simulink model "Template_v3_08_2022a_Jetson"  (R2022a)
settings: Solver=FixedStepAuto  StartTime=0.0  StopTime=tsim  FixedStep=baseRate  RelTol=1e-3  EnableMultiTasking=on
values from neighbouring files (symbols this model uses):
  baseRate = 0.05    [Run_Initializer.m]
  drop_states_ARM = [ pi/2, pi/2, 0]    [Run_Initializer.m]
  drop_states_BLACK = [ xLength/2, yLength/2, 0]    [Run_Initializer.m]
  drop_states_BLUE = [ xLength/2-0.5; yLength/2; 0]    [Run_Initializer.m]
  drop_states_RED = [ xLength/2+0.5, yLength/2, pi]    [Run_Initializer.m]
  F_Black_X_nominal = 0.2196    [Run_Initializer.m]
  F_Black_Y_nominal = 0.2825    [Run_Initializer.m]
  F_Blue_X_nominal = 0.2196    [Run_Initializer.m]
  F_Blue_Y_nominal = 0.2825    [Run_Initializer.m]
  F_red_X_nominal = 0.2196    [Run_Initializer.m]
  F_red_Y_nominal = 0.2825    [Run_Initializer.m]
  F_thrusters_BLACK = [F_Black_X_nominal; F_Black_X_nominal;                             F_Black_Y_nominal; F_Black_Y_nominal; F_Black_X_nominal;                              F_Black_X_nominal; F_Black_Y_nominal; F_Black_Y_nominal]    [Run_Initializer.m]
  F_thrusters_BLUE = [F_Blue_X_nominal; F_Blue_X_nominal;                             F_Blue_Y_nominal; F_Blue_Y_nominal; F_Blue_X_nominal;                              F_Blue_X_nominal; F_Blue_Y_nominal; F_Blue_Y_nominal]    [Run_Initializer.m]
  F_thrusters_RED = [F_red_X_nominal; F_red_X_nominal;                             F_red_Y_nominal; F_red_Y_nominal; F_red_X_nominal;                              F_red_X_nominal; F_red_Y_nominal; F_red_Y_nominal]    [Run_Initializer.m]
  Gamma1 = 0.0025    [Run_Initializer.m]
  Gamma2 = 100    [Run_Initializer.m]
  Gamma3 = 10    [Run_Initializer.m]
  Gamma4 = 0.001    [Run_Initializer.m]
  Gamma5 = 100    [Run_Initializer.m]
  Gamma6 = 0.001    [Run_Initializer.m]
  home_states_BLACK = [ xLength/2; yLength/2; 0]    [Run_Initializer.m]
  home_states_BLUE = [ xLength/2-0.9; yLength/2; 0]    [Run_Initializer.m]
  home_states_RED = [ xLength/2+0.9; yLength/2; pi]    [Run_Initializer.m]
  init_states_BLACK = [ xLength/2; yLength/2; 0]    [Run_Initializer.m]
  init_states_BLUE = [ xLength/2-0.9; yLength/2; 0]    [Run_Initializer.m]
  init_states_RED = [ xLength/2+0.9; yLength/2; pi]    [Run_Initializer.m]
  Kd_elarm = 0.05    [Run_Initializer.m]
  Kd_sharm = 0.05    [Run_Initializer.m]
  Kd_tb = 0.4    [Run_Initializer.m]
  Kd_tblue = 0.4    [Run_Initializer.m]
  Kd_tr = 0.4    [Run_Initializer.m]
  Kd_wrarm = 0.005    [Run_Initializer.m]
  Kd_xb = 8    [Run_Initializer.m]
  Kd_xblue = 8    [Run_Initializer.m]
  Kd_xr = 8    [Run_Initializer.m]
  Kd_yb = 8    [Run_Initializer.m]
  Kd_yblue = 8    [Run_Initializer.m]
  Kd_yr = 8    [Run_Initializer.m]
  Kp = [0.08 0 0 ... (first row only)    [Run_Initializer.m]
  Kp_elarm = 0.08    [Run_Initializer.m]
  Kp_sharm = 0.15    [Run_Initializer.m]
  Kp_tb = 0.1    [Run_Initializer.m]
  Kp_tblue = 0.1    [Run_Initializer.m]
  Kp_tr = 0.1    [Run_Initializer.m]
  Kp_wrarm = 0.007    [Run_Initializer.m]
  Kp_xb = 2    [Run_Initializer.m]
  Kp_xblue = 2    [Run_Initializer.m]
  Kp_xr = 2    [Run_Initializer.m]
  Kp_yb = 2    [Run_Initializer.m]
  Kp_yblue = 2    [Run_Initializer.m]
  Kp_yr = 2    [Run_Initializer.m]
  Kv = [0.05 0 0 ... (first row only)    [Run_Initializer.m]
  noise_variance_BLACK = 0    [Run_Initializer.m]
  noise_variance_BLUE = 0    [Run_Initializer.m]
  noise_variance_RED = 0    [Run_Initializer.m]
  Phase0_End = Phase0_Duration    (= 10)    [Run_Initializer.m]
  Phase1_End = Phase0_Duration + Phase1_Duration    (= 15)    [Run_Initializer.m]
  Phase2_End = Phase0_Duration + Phase1_Duration +                                   Phase2_Duration    (= 35)    [Run_Initializer.m]
  Phase3_End = Phase0_Duration + Phase1_Duration +                                   Phase2_Duration + Phase3_Duration    (= 550)    [Run_Initializer.m]
  Phase3_SubPhase1_End = Phase2_End + Phase3_SubPhase1_Duration    (= 155)    [Run_Initializer.m]
  Phase3_SubPhase2_End = Phase2_End + Phase3_SubPhase1_Duration +                                   Phase3_SubPhase2_Duration    (= 165)    [Run_Initializer.m]
  Phase3_SubPhase3_End = Phase2_End + Phase3_SubPhase1_Duration +                                   Phase3_SubPhase2_Duration +                                  Phase3_SubPhase3_Duration    (= 195)    [Run_Initializer.m]
  Phase3_SubPhase4_End = Phase2_End + Phase3_SubPhase1_Duration +                                   Phase3_SubPhase2_Duration +                                  Phase3_SubPhase3_Duration +                                  Phase3_SubPhase4_Duration    [Run_Initializer.m]
  Phase4_End = Phase0_Duration + Phase1_Duration +                                   Phase2_Duration + Phase3_Duration +                                   Phase4_Duration    (= 670)    [Run_Initializer.m]
  Phase5_End = Phase0_Duration + Phase1_Duration +                                   Phase2_Duration + Phase3_Duration +                                   Phase4_Duration + Phase5_Duration    (= 690)    [Run_Initializer.m]
  thruster_dist2CG_BLACK = [83.42;-52.58;55.94;-60.05;54.08;-53.92;77.06;-55.94]    [Run_Initializer.m]
  thruster_dist2CG_BLUE = [73.54;-64.46;81.39;-60.11;64.46;-65.94;54.61;-74.39]    [Run_Initializer.m]
  thruster_dist2CG_RED = [49.92;-78.08;70.46;-63.54;81.08;-50.42;57.44;-75.96]    [Run_Initializer.m]
  Tz_lim_elarm = .1    (= 0.1)    [Run_Initializer.m]
  Tz_lim_sharm = .1    (= 0.1)    [Run_Initializer.m]
  Tz_lim_wrarm = .1    (= 0.1)    [Run_Initializer.m]
  xLength = 3.51155    [Run_Initializer.m]
  yLength = 2.41935    [Run_Initializer.m]
undefined symbols (not defined in the file or in its folder): DiscIntNeverNeededParam, model_param, platformSelection, serverRate, simMode
libraries: dspstat3 x18, raspberrypiBasiclib x10, MainLibrary x6, dspsigops x6, simulink x6, embedlinuxBasiclib x5, mspfiltlib x3, dsparch4 x3, nvidiaBasiclib x2, nvidiaSharedBlocks x1, sensehatlib x1
(part 5 of 14)

== system Template_v3_08_2022a_Jetson/IMU Data and Algorithms/Change BLACK Behavior/Fix Initial Bias ==
  Actual Gyro : Inport
  Correct GyroX : Subsystem
  Correct GyroY : Subsystem
  Correct GyroZ : Subsystem
  Demux : Demux  Outputs=3
  Mux : Mux  Inputs=3
  Corrected Gyro : Outport  VectorParamsAs1DForOutWhenUnconnected=off
  wires:
  Demux/1 -> Correct GyroX/1(In1)
  Demux/2 -> Correct GyroY/1(In1)
  Demux/3 -> Correct GyroZ/1(In1)
  Correct GyroX/1(Out1) -> Mux/1
  Correct GyroY/1(Out1) -> Mux/2
  Correct GyroZ/1(Out1) -> Mux/3
  Mux/1 -> Corrected Gyro/1
  Actual Gyro/1 -> Demux/1

== system Template_v3_08_2022a_Jetson/IMU Data and Algorithms/Change BLACK Behavior/Fix Initial Bias (Accel) ==
  Actual Accel : Inport
  Correct AccelX : Subsystem
  Correct AccelY : Subsystem
  Correct AccelZ : Subsystem
  Demux : Demux  Outputs=3
  Mux : Mux  Inputs=3
  Corrected Accel : Outport  VectorParamsAs1DForOutWhenUnconnected=off
  wires:
  Demux/1 -> Correct AccelX/1(In1)
  Demux/2 -> Correct AccelY/1(In1)
  Demux/3 -> Correct AccelZ/1(In1)
  Correct AccelX/1(Out1) -> Mux/1
  Correct AccelY/1(Out1) -> Mux/2
  Correct AccelZ/1(Out1) -> Mux/3
  Mux/1 -> Corrected Accel/1
  Actual Accel/1 -> Demux/1

== system Template_v3_08_2022a_Jetson/IMU Data and Algorithms/Change BLUE Behavior/Fix Initial Bias ==
  Actual Gyro : Inport
  Correct GyroX : Subsystem
  Correct GyroY : Subsystem
  Correct GyroZ : Subsystem
  Demux : Demux  Outputs=3
  Mux : Mux  Inputs=3
  Corrected Gyro : Outport  VectorParamsAs1DForOutWhenUnconnected=off
  wires:
  Demux/1 -> Correct GyroX/1(In1)
  Demux/2 -> Correct GyroY/1(In1)
  Demux/3 -> Correct GyroZ/1(In1)
  Correct GyroX/1(Out1) -> Mux/1
  Correct GyroY/1(Out1) -> Mux/2
  Correct GyroZ/1(Out1) -> Mux/3
  Mux/1 -> Corrected Gyro/1
  Actual Gyro/1 -> Demux/1

== system Template_v3_08_2022a_Jetson/IMU Data and Algorithms/Change BLUE Behavior/Fix Initial Bias (Accel) ==
  Actual Accel : Inport
  Correct AccelX : Subsystem
  Correct AccelY : Subsystem
  Correct AccelZ : Subsystem
  Demux : Demux  Outputs=3
  Mux : Mux  Inputs=3
  Corrected Accel : Outport  VectorParamsAs1DForOutWhenUnconnected=off
  wires:
  Demux/1 -> Correct AccelX/1(In1)
  Demux/2 -> Correct AccelY/1(In1)
  Demux/3 -> Correct AccelZ/1(In1)
  Correct AccelX/1(Out1) -> Mux/1
  Correct AccelY/1(Out1) -> Mux/2
  Correct AccelZ/1(Out1) -> Mux/3
  Mux/1 -> Corrected Accel/1
  Actual Accel/1 -> Demux/1

== system Template_v3_08_2022a_Jetson/IMU Data and Algorithms/Change RED Behavior/Fix Initial Bias ==
  Actual Gyro : Inport
  Correct GyroX : Subsystem
  Correct GyroY : Subsystem
  Correct GyroZ : Subsystem
  Demux : Demux  Outputs=3
  Mux : Mux  Inputs=3
  Corrected Gyro : Outport  VectorParamsAs1DForOutWhenUnconnected=off
  wires:
  Demux/1 -> Correct GyroX/1(In1)
  Demux/2 -> Correct GyroY/1(In1)
  Demux/3 -> Correct GyroZ/1(In1)
  Correct GyroX/1(Out1) -> Mux/1
  Correct GyroY/1(Out1) -> Mux/2
  Correct GyroZ/1(Out1) -> Mux/3
  Mux/1 -> Corrected Gyro/1
  Actual Gyro/1 -> Demux/1

== system Template_v3_08_2022a_Jetson/IMU Data and Algorithms/Change RED Behavior/Fix Initial Bias (Accel) ==
  Actual Accel : Inport
  Correct AccelX : Subsystem
  Correct AccelY : Subsystem
  Correct AccelZ : Subsystem
  Demux : Demux  Outputs=3
  Mux : Mux  Inputs=3
  Corrected Accel : Outport  VectorParamsAs1DForOutWhenUnconnected=off
  wires:
  Demux/1 -> Correct AccelX/1(In1)
  Demux/2 -> Correct AccelY/1(In1)
  Demux/3 -> Correct AccelZ/1(In1)
  Correct AccelX/1(Out1) -> Mux/1
  Correct AccelY/1(Out1) -> Mux/2
  Correct AccelZ/1(Out1) -> Mux/3
  Mux/1 -> Corrected Accel/1
  Actual Accel/1 -> Demux/1

== system Template_v3_08_2022a_Jetson/Manipulator Encoder Data/Change Behavior/Correct for dropouts ==
  In1 : Inport
  Correct Dropouts : MATLAB Function  TreatAsAtomicUnit=on
  Delay1 : Delay  DelayLength=1  InitialCondition=0
  Delay2 : Delay  InitialCondition=0
  Delay3 : Delay  DelayLength=4  InitialCondition=0
  Delay4 : Delay  DelayLength=5  InitialCondition=0
  Delay5 : Delay  DelayLength=3  InitialCondition=0
  Mux : Mux  Inputs=6
  FixedInput : Outport
  wires:
  Correct Dropouts/1(FixedInput) -> FixedInput/1
  In1/1 -> Mux/1, Delay1/1, Delay2/1, Delay4/1, Delay3/1, Delay5/1
  Delay1/1 -> Mux/2
  Delay2/1 -> Mux/3
  Delay5/1 -> Mux/4
  Delay3/1 -> Mux/5
  Delay4/1 -> Mux/6
  Mux/1 -> Correct Dropouts/1(InputRaw)

== system Template_v3_08_2022a_Jetson/Manipulator Encoder Data/Change Behavior/Correct for dropouts1 ==
  In1 : Inport
  Correct Dropouts : MATLAB Function  TreatAsAtomicUnit=on
  Delay1 : Delay  DelayLength=1  InitialCondition=0
  Delay2 : Delay  InitialCondition=0
  Delay3 : Delay  DelayLength=4  InitialCondition=0
  Delay4 : Delay  DelayLength=5  InitialCondition=0
  Delay5 : Delay  DelayLength=3  InitialCondition=0
  Mux : Mux  Inputs=6
  FixedInput : Outport
  wires:
  Correct Dropouts/1(FixedInput) -> FixedInput/1
  In1/1 -> Mux/1, Delay1/1, Delay2/1, Delay4/1, Delay3/1, Delay5/1
  Delay1/1 -> Mux/2
  Delay2/1 -> Mux/3
  Delay5/1 -> Mux/4
  Delay3/1 -> Mux/5
  Delay4/1 -> Mux/6
  Mux/1 -> Correct Dropouts/1(InputRaw)

== system Template_v3_08_2022a_Jetson/Manipulator Encoder Data/Change Behavior/Correct for dropouts2 ==
  In1 : Inport
  Correct Dropouts : MATLAB Function  TreatAsAtomicUnit=on
  Delay1 : Delay  DelayLength=1  InitialCondition=0
  Delay2 : Delay  InitialCondition=0
  Delay3 : Delay  DelayLength=4  InitialCondition=0
  Delay4 : Delay  DelayLength=5  InitialCondition=0
  Delay5 : Delay  DelayLength=3  InitialCondition=0
  Mux : Mux  Inputs=6
  FixedInput : Outport
  wires:
  Correct Dropouts/1(FixedInput) -> FixedInput/1
  In1/1 -> Mux/1, Delay1/1, Delay2/1, Delay4/1, Delay3/1, Delay5/1
  Delay1/1 -> Mux/2
  Delay2/1 -> Mux/3
  Delay5/1 -> Mux/4
  Delay3/1 -> Mux/5
  Delay4/1 -> Mux/6
  Mux/1 -> Correct Dropouts/1(InputRaw)

== system Template_v3_08_2022a_Jetson/Phase #2: Move to Initial Position/Change BLACK Behavior/Custom Discrete PD (Attitude) ==
  ez : Inport
  Sum3 : Sum
  kd_tb : Gain  Gain=Kd_tb
  kp_tb : Gain  Gain=Kp_tb
  "x_dot -> x1" : Subsystem
  Tz : Outport  VectorParamsAs1DForOutWhenUnconnected=off
  wires:
  kd_tb/1 -> Sum3/1
  Sum3/1 -> Tz/1
  kp_tb/1 -> Sum3/2
  "x_dot -> x1"/1(dy(t)/dt) -> kd_tb/1
  ez/1 -> "x_dot -> x1"/1(y(t)), kp_tb/1

== system Template_v3_08_2022a_Jetson/Phase #2: Move to Initial Position/Change BLACK Behavior/Custom Discrete PD (X-Position) ==
  ex : Inport
  Sum3 : Sum
  kd_xb : Gain  Gain=Kd_xb
  kp_xb : Gain  Gain=Kp_xb
  "x_dot -> x1" : Subsystem
  Fx : Outport  VectorParamsAs1DForOutWhenUnconnected=off
  wires:
  kd_xb/1 -> Sum3/1
  ex/1 -> "x_dot -> x1"/1(y(t)), kp_xb/1
  kp_xb/1 -> Sum3/2
  "x_dot -> x1"/1(dy(t)/dt) -> kd_xb/1
  Sum3/1 -> Fx/1

== system Template_v3_08_2022a_Jetson/Phase #2: Move to Initial Position/Change BLACK Behavior/Custom Discrete PD (Y-Position) ==
  ey : Inport
  Sum3 : Sum
  kd_yb : Gain  Gain=Kd_yb
  kp_yb : Gain  Gain=Kp_yb
  "x_dot -> x1" : Subsystem
  Fy : Outport  VectorParamsAs1DForOutWhenUnconnected=off
  wires:
  kd_yb/1 -> Sum3/1
  Sum3/1 -> Fy/1
  kp_yb/1 -> Sum3/2
  "x_dot -> x1"/1(dy(t)/dt) -> kd_yb/1
  ey/1 -> "x_dot -> x1"/1(y(t)), kp_yb/1

== system Template_v3_08_2022a_Jetson/Phase #2: Move to Initial Position/Change BLACK Behavior/Hough Control ==
  Ref : Inport
  Act : Inport  Port=2
  MATLAB Function2 : MATLAB Function  TreatAsAtomicUnit=on
  MATLAB Function3 : MATLAB Function  TreatAsAtomicUnit=on
  MATLAB Function4 : MATLAB Function  TreatAsAtomicUnit=on
  Subtract2 : Sum  Inputs=+-
  Err : Outport  VectorParamsAs1DForOutWhenUnconnected=off
  wires:
  MATLAB Function4/1(e_out) -> Err/1
  MATLAB Function2/1(Oy) -> MATLAB Function4/1(Oy)
  Subtract2/1 -> MATLAB Function4/2(e_in)
  MATLAB Function2/2(Ox) -> Subtract2/1
  Act/1 -> MATLAB Function3/1(z)
  Ref/1 -> MATLAB Function2/1(z)
  MATLAB Function3/1(Ox) -> Subtract2/2

== system Template_v3_08_2022a_Jetson/Phase #2: Move to Initial Position/Change BLUE Behavior/Custom Discrete PD (Attitude) ==
  ez : Inport
  Sum3 : Sum
  kd_tb : Gain  Gain=Kd_tblue
  kp_tb : Gain  Gain=Kp_tblue
  "x_dot -> x1" : Subsystem
  Tz : Outport  VectorParamsAs1DForOutWhenUnconnected=off
  wires:
  kd_tb/1 -> Sum3/1
  Sum3/1 -> Tz/1
  kp_tb/1 -> Sum3/2
  "x_dot -> x1"/1(dy(t)/dt) -> kd_tb/1
  ez/1 -> "x_dot -> x1"/1(y(t)), kp_tb/1

== system Template_v3_08_2022a_Jetson/Phase #2: Move to Initial Position/Change BLUE Behavior/Custom Discrete PD (X-Position) ==
  ex : Inport
  Sum3 : Sum
  kd_xb : Gain  Gain=Kd_xblue
  kp_xb : Gain  Gain=Kp_xblue
  "x_dot -> x1" : Subsystem
  Fx : Outport  VectorParamsAs1DForOutWhenUnconnected=off
  wires:
  kd_xb/1 -> Sum3/1
  ex/1 -> "x_dot -> x1"/1(y(t)), kp_xb/1
  kp_xb/1 -> Sum3/2
  "x_dot -> x1"/1(dy(t)/dt) -> kd_xb/1
  Sum3/1 -> Fx/1

== system Template_v3_08_2022a_Jetson/Phase #2: Move to Initial Position/Change BLUE Behavior/Custom Discrete PD (Y-Position) ==
  ey : Inport
  Sum3 : Sum
  kd_yb : Gain  Gain=Kd_yblue
  kp_yb : Gain  Gain=Kp_yblue
  "x_dot -> x1" : Subsystem
  Fy : Outport  VectorParamsAs1DForOutWhenUnconnected=off
  wires:
  kd_yb/1 -> Sum3/1
  Sum3/1 -> Fy/1
  kp_yb/1 -> Sum3/2
  "x_dot -> x1"/1(dy(t)/dt) -> kd_yb/1
  ey/1 -> "x_dot -> x1"/1(y(t)), kp_yb/1

== system Template_v3_08_2022a_Jetson/Phase #2: Move to Initial Position/Change BLUE Behavior/Hough Control ==
  Ref : Inport
  Act : Inport  Port=2
  MATLAB Function2 : MATLAB Function  TreatAsAtomicUnit=on
  MATLAB Function3 : MATLAB Function  TreatAsAtomicUnit=on
  MATLAB Function4 : MATLAB Function  TreatAsAtomicUnit=on
  Subtract2 : Sum  Inputs=+-
  Err : Outport  VectorParamsAs1DForOutWhenUnconnected=off
  wires:
  MATLAB Function4/1(e_out) -> Err/1
  MATLAB Function2/1(Oy) -> MATLAB Function4/1(Oy)
  Subtract2/1 -> MATLAB Function4/2(e_in)
  MATLAB Function2/2(Ox) -> Subtract2/1
  Act/1 -> MATLAB Function3/1(z)
  Ref/1 -> MATLAB Function2/1(z)
  MATLAB Function3/1(Ox) -> Subtract2/2

== system Template_v3_08_2022a_Jetson/Phase #2: Move to Initial Position/Change RED Behavior/Custom Discrete PD (Attitude) ==
  ez : Inport
  Sum3 : Sum
  kd_tr : Gain  Gain=Kd_tr
  kp_tr : Gain  Gain=Kp_tr
  "x_dot -> x2" : Subsystem
  Tz : Outport  VectorParamsAs1DForOutWhenUnconnected=off
  wires:
  kd_tr/1 -> Sum3/1
  Sum3/1 -> Tz/1
  kp_tr/1 -> Sum3/2
  "x_dot -> x2"/1(dy(t)/dt) -> kd_tr/1
  ez/1 -> "x_dot -> x2"/1(y(t)), kp_tr/1

== system Template_v3_08_2022a_Jetson/Phase #2: Move to Initial Position/Change RED Behavior/Custom Discrete PD (X-Position) ==
  ex : Inport
  Sum3 : Sum
  kd_xr : Gain  Gain=Kd_xr
  kp_xr : Gain  Gain=Kp_xr
  "x_dot -> x2" : Subsystem
  Fx : Outport  VectorParamsAs1DForOutWhenUnconnected=off
  wires:
  kd_xr/1 -> Sum3/1
  ex/1 -> "x_dot -> x2"/1(y(t)), kp_xr/1
  kp_xr/1 -> Sum3/2
  "x_dot -> x2"/1(dy(t)/dt) -> kd_xr/1
  Sum3/1 -> Fx/1

== system Template_v3_08_2022a_Jetson/Phase #2: Move to Initial Position/Change RED Behavior/Custom Discrete PD (Y-Position) ==
  ey : Inport
  Sum3 : Sum
  kd_yr : Gain  Gain=Kd_yr
  kp_yr : Gain  Gain=Kp_yr
  "x_dot -> x2" : Subsystem
  Fy : Outport  VectorParamsAs1DForOutWhenUnconnected=off
  wires:
  kd_yr/1 -> Sum3/1
  Sum3/1 -> Fy/1
  kp_yr/1 -> Sum3/2
  "x_dot -> x2"/1(dy(t)/dt) -> kd_yr/1
  ey/1 -> "x_dot -> x2"/1(y(t)), kp_yr/1

== system Template_v3_08_2022a_Jetson/Phase #2: Move to Initial Position/Change RED Behavior/Hough Control ==
  Ref : Inport
  Act : Inport  Port=2
  MATLAB Function2 : MATLAB Function  TreatAsAtomicUnit=on
  MATLAB Function3 : MATLAB Function  TreatAsAtomicUnit=on
  MATLAB Function4 : MATLAB Function  TreatAsAtomicUnit=on
  Subtract2 : Sum  Inputs=+-
  Err : Outport  VectorParamsAs1DForOutWhenUnconnected=off
  wires:
  MATLAB Function4/1(e_out) -> Err/1
  MATLAB Function2/1(Oy) -> MATLAB Function4/1(Oy)
  Subtract2/1 -> MATLAB Function4/2(e_in)
  MATLAB Function2/2(Ox) -> Subtract2/1
  Act/1 -> MATLAB Function3/1(z)
  Ref/1 -> MATLAB Function2/1(z)
  MATLAB Function3/1(Ox) -> Subtract2/2

== system Template_v3_08_2022a_Jetson/Phase #2: Move to Initial Position/Change RED Behavior/RED ==
  note: ARM Control Law - RED
  note: When the ARM is not in use, send zeros.
  Action Port : ActionPort  ActionPortLabel=else
  Constant7 : Constant  Value=0
  RED_Fx1 : DataStoreWrite  DataStoreName=RED_Tz_Shoulder  IndexOptions=Index vector (dialog)  Indices=1  OutputSizes=1
  RED_Fy1 : DataStoreWrite  DataStoreName=RED_Tz_Elbow  IndexOptions=Index vector (dialog)  Indices=1  OutputSizes=1
  RED_Tz1 : DataStoreWrite  DataStoreName=RED_Tz_Wrist  IndexOptions=Index vector (dialog)  Indices=1  OutputSizes=1
  wires:
  Constant7/1 -> RED_Fx1/1, RED_Fy1/1, RED_Tz1/1

== system Template_v3_08_2022a_Jetson/Phase #2: Move to Initial Position/Change RED Behavior/RED+ARM ==
  note: ARM Control Law - RED
  note: This section is reserved for any control law for the robotic manipulator.
  Action Port : ActionPort  ActionPortLabel=if(u1 == 4 | u1 == 5 | u1 == 10 | u1 == 11)
  ARM_EL_Rz : DataStoreRead  DataStoreName=RED_Rz_Elbow  IndexOptions=Index vector (dialog)  Indices=1  OutputSizes=1
  ARM_EL_Tz : DataStoreWrite  DataStoreName=RED_Tz_Elbow  IndexOptions=Index vector (dialog)  Indices=1  OutputSizes=1
  ARM_SH_Rz : DataStoreRead  DataStoreName=RED_Rz_Shoulder  IndexOptions=Index vector (dialog)  Indices=1  OutputSizes=1
  ARM_SH_Tz : DataStoreWrite  DataStoreName=RED_Tz_Shoulder  IndexOptions=Index vector (dialog)  Indices=1  OutputSizes=1
  ARM_WR_Rz : DataStoreRead  DataStoreName=RED_Rz_Wrist  IndexOptions=Index vector (dialog)  Indices=1  OutputSizes=1
  ARM_WR_Tz : DataStoreWrite  DataStoreName=RED_Tz_Wrist  IndexOptions=Index vector (dialog)  Indices=1  OutputSizes=1
  Constant7 : Constant  Value=0
  Constant8 : Constant  Value=pi/2
  Constant9 : Constant  Value=pi/2
  Custom Discrete PD (Elbow) : Subsystem
  Custom Discrete PD (Shoulder) : Subsystem
  Custom Discrete PD (Wrist) : Subsystem
  Saturation : Saturate  UpperLimit=Tz_lim_sharm  LowerLimit=-Tz_lim_sharm
  Saturation1 : Saturate  UpperLimit=Tz_lim_elarm  LowerLimit=-Tz_lim_elarm
  Saturation3 : Saturate  UpperLimit=Tz_lim_wrarm  LowerLimit=-Tz_lim_wrarm
  Subtract2 : Sum  Inputs=+-
  Subtract3 : Sum  Inputs=+-
  Subtract4 : Sum  Inputs=+-
  wires:
  Saturation3/1 -> ARM_WR_Tz/1
  Custom Discrete PD (Elbow)/1(Fy) -> Saturation1/1
  Saturation1/1 -> ARM_EL_Tz/1
  Constant9/1 -> Subtract3/1
  Subtract3/1 -> Custom Discrete PD (Elbow)/1(ey)
  ARM_EL_Rz/1 -> Subtract3/2
  ARM_WR_Rz/1 -> Subtract4/2
  Custom Discrete PD (Shoulder)/1(Fx) -> Saturation/1
  Constant8/1 -> Subtract2/1
  Custom Discrete PD (Wrist)/1(Fy) -> Saturation3/1
  Constant7/1 -> Subtract4/1
  Subtract4/1 -> Custom Discrete PD (Wrist)/1(ey)
  Saturation/1 -> ARM_SH_Tz/1
  ARM_SH_Rz/1 -> Subtract2/2
  Subtract2/1 -> Custom Discrete PD (Shoulder)/1(ex)

== system Template_v3_08_2022a_Jetson/Phase #3: Experiment/Change BLACK Behavior/Sub-Phase #1 ==
  note: PD Control Law - BLACK
  note: Additional Blocks
  note: A simple PD control law is used here to command the platform to it's initial position, as defined in the initializer.
  note: Additional blocks are stored here.
  Action Port : ActionPort  ActionPortLabel=if(u1 < u2)
  BLACK_Fx : DataStoreWrite  DataStoreName=BLACK_Fx  IndexOptions=Index vector (dialog)  Indices=1  OutputSizes=1
  BLACK_Fy : DataStoreWrite  DataStoreName=BLACK_Fy  IndexOptions=Index vector (dialog)  Indices=1  OutputSizes=1
  BLACK_Px : DataStoreRead  DataStoreName=BLACK_Px  IndexOptions=Index vector (dialog)  Indices=1  OutputSizes=1
  "BLACK_Py " : DataStoreRead  DataStoreName=BLACK_Py  IndexOptions=Index vector (dialog)  Indices=1  OutputSizes=1
  BLACK_Rz : DataStoreRead  DataStoreName=BLACK_Rz  IndexOptions=Index vector (dialog)  Indices=1  OutputSizes=1
  BLACK_RzD1 : Subsystem
  BLACK_Tz : DataStoreWrite  DataStoreName=BLACK_Tz  IndexOptions=Index vector (dialog)  Indices=1  OutputSizes=1
  Custom Discrete PD (Attitude) : Subsystem
  Custom Discrete PD (X-Position) : Subsystem
  Custom Discrete PD (Y-Position) : Subsystem
  Data Store Write3 : DataStoreWrite  DataStoreName=Float_State  IndexOptions=Index vector (dialog)  Indices=1  OutputSizes=1
  Desired X-Position (BLACK) : Constant  Value=xLength/2  SampleTime=-1
  Desired Y-Position (BLACK) : Constant  Value=yLength/2  SampleTime=-1
  Hough Control : Subsystem
  Puck State : Constant
  Subtract : Sum  Inputs=+-
  Subtract1 : Sum  Inputs=+-
  wires:
  Puck State/1 -> Data Store Write3/1
  "BLACK_Py "/1 -> Subtract1/2
  Desired X-Position (BLACK)/1 -> Subtract/1
  BLACK_RzD1/1(Out1) -> Hough Control/1(Ref)
  Custom Discrete PD (X-Position)/1(Fx) -> BLACK_Fx/1
  Desired Y-Position (BLACK)/1 -> Subtract1/1
  Hough Control/1(Err) -> Custom Discrete PD (Attitude)/1(ez)
  Subtract/1 -> Custom Discrete PD (X-Position)/1(ex)
  Custom Discrete PD (Y-Position)/1(Fy) -> BLACK_Fy/1
  Subtract1/1 -> Custom Discrete PD (Y-Position)/1(ey)
  Custom Discrete PD (Attitude)/1(Tz) -> BLACK_Tz/1
  BLACK_Rz/1 -> Hough Control/2(Act)
  BLACK_Px/1 -> Subtract/2

== system Template_v3_08_2022a_Jetson/Phase #3: Experiment/Change BLACK Behavior/Sub-Phase #2  ==
  note: PD Control Law - BLACK
  note: Additional Blocks
  note: Additional blocks are stored here.
  Action Port : ActionPort  ActionPortLabel=elseif(u1 < u3)
  BLACK_Fx : DataStoreWrite  DataStoreName=BLACK_Fx  IndexOptions=Index vector (dialog)  Indices=1  OutputSizes=1
  BLACK_Fy : DataStoreWrite  DataStoreName=BLACK_Fy  IndexOptions=Index vector (dialog)  Indices=1  OutputSizes=1
  BLACK_Px : DataStoreRead  DataStoreName=BLACK_Px  IndexOptions=Index vector (dialog)  Indices=1  OutputSizes=1
  "BLACK_Py " : DataStoreRead  DataStoreName=BLACK_Py  IndexOptions=Index vector (dialog)  Indices=1  OutputSizes=1
  BLACK_Rz : DataStoreRead  DataStoreName=BLACK_Rz  IndexOptions=Index vector (dialog)  Indices=1  OutputSizes=1
  BLACK_RzD1 : Subsystem
  BLACK_Tz : DataStoreWrite  DataStoreName=BLACK_Tz  IndexOptions=Index vector (dialog)  Indices=1  OutputSizes=1
  Custom Discrete PD (Attitude) : Subsystem
  Custom Discrete PD (X-Position) : Subsystem
  Custom Discrete PD (Y-Position) : Subsystem
  Data Store Write3 : DataStoreWrite  DataStoreName=Float_State  IndexOptions=Index vector (dialog)  Indices=1  OutputSizes=1
  Desired X-Position (BLACK) : Constant  Value=xLength/2  SampleTime=-1
  Desired Y-Position (BLACK) : Constant  Value=yLength/2  SampleTime=-1
  Hough Control : Subsystem
  Puck State : Constant
  Subtract : Sum  Inputs=+-
  Subtract1 : Sum  Inputs=+-
  wires:
  Puck State/1 -> Data Store Write3/1
  BLACK_Px/1 -> Subtract/2
  Custom Discrete PD (Y-Position)/1(Fy) -> BLACK_Fy/1
  Subtract/1 -> Custom Discrete PD (X-Position)/1(ex)
  Desired Y-Position (BLACK)/1 -> Subtract1/1
  Custom Discrete PD (Attitude)/1(Tz) -> BLACK_Tz/1
  Subtract1/1 -> Custom Discrete PD (Y-Position)/1(ey)
  BLACK_Rz/1 -> Hough Control/2(Act)
  Custom Discrete PD (X-Position)/1(Fx) -> BLACK_Fx/1
  Hough Control/1(Err) -> Custom Discrete PD (Attitude)/1(ez)
  "BLACK_Py "/1 -> Subtract1/2
  Desired X-Position (BLACK)/1 -> Subtract/1
  BLACK_RzD1/1(Out1) -> Hough Control/1(Ref)

== system Template_v3_08_2022a_Jetson/Phase #3: Experiment/Change BLACK Behavior/Sub-Phase #3  ==
  note: PD Control Law - BLACK
  note: Additional Blocks
  note: Additional blocks are stored here.
  Action Port : ActionPort  ActionPortLabel=elseif( u1 < u4)
  BLACK_Fx : DataStoreWrite  DataStoreName=BLACK_Fx  IndexOptions=Index vector (dialog)  Indices=1  OutputSizes=1
  BLACK_Fy : DataStoreWrite  DataStoreName=BLACK_Fy  IndexOptions=Index vector (dialog)  Indices=1  OutputSizes=1
  BLACK_Px : DataStoreRead  DataStoreName=BLACK_Px  IndexOptions=Index vector (dialog)  Indices=1  OutputSizes=1
  "BLACK_Py " : DataStoreRead  DataStoreName=BLACK_Py  IndexOptions=Index vector (dialog)  Indices=1  OutputSizes=1
  BLACK_Rz : DataStoreRead  DataStoreName=BLACK_Rz  IndexOptions=Index vector (dialog)  Indices=1  OutputSizes=1
  BLACK_RzD1 : Subsystem
  BLACK_Tz : DataStoreWrite  DataStoreName=BLACK_Tz  IndexOptions=Index vector (dialog)  Indices=1  OutputSizes=1
  Custom Discrete PD (Attitude) : Subsystem
  Custom Discrete PD (X-Position) : Subsystem
  Custom Discrete PD (Y-Position) : Subsystem
  Data Store Write3 : DataStoreWrite  DataStoreName=Float_State  IndexOptions=Index vector (dialog)  Indices=1  OutputSizes=1
  Desired X-Position (BLACK) : Constant  Value=xLength/2  SampleTime=-1
  Desired Y-Position (BLACK) : Constant  Value=yLength/2  SampleTime=-1
  Hough Control : Subsystem
  Puck State : Constant
  Subtract : Sum  Inputs=+-
  Subtract1 : Sum  Inputs=+-
  wires:
  Puck State/1 -> Data Store Write3/1
  BLACK_Px/1 -> Subtract/2
  Custom Discrete PD (Y-Position)/1(Fy) -> BLACK_Fy/1
  Subtract/1 -> Custom Discrete PD (X-Position)/1(ex)
  Desired Y-Position (BLACK)/1 -> Subtract1/1
  Custom Discrete PD (Attitude)/1(Tz) -> BLACK_Tz/1
  Subtract1/1 -> Custom Discrete PD (Y-Position)/1(ey)
  BLACK_Rz/1 -> Hough Control/2(Act)
  Custom Discrete PD (X-Position)/1(Fx) -> BLACK_Fx/1
  Hough Control/1(Err) -> Custom Discrete PD (Attitude)/1(ez)
  "BLACK_Py "/1 -> Subtract1/2
  Desired X-Position (BLACK)/1 -> Subtract/1
  BLACK_RzD1/1(Out1) -> Hough Control/1(Ref)

== system Template_v3_08_2022a_Jetson/Phase #3: Experiment/Change BLACK Behavior/Sub-Phase #4 ==
  note: PD Control Law - BLACK
  note: Additional Blocks
  note: A simple PD control law is used here to command the platform to it's initial position, as defined in the initializer.
  note: Additional blocks are stored here.
  Action Port : ActionPort  ActionPortLabel=elseif( u1 < u5)
  BLACK_Fx : DataStoreWrite  DataStoreName=BLACK_Fx  IndexOptions=Index vector (dialog)  Indices=1  OutputSizes=1
  BLACK_Fy : DataStoreWrite  DataStoreName=BLACK_Fy  IndexOptions=Index vector (dialog)  Indices=1  OutputSizes=1
  BLACK_Px : DataStoreRead  DataStoreName=BLACK_Px  IndexOptions=Index vector (dialog)  Indices=1  OutputSizes=1
  "BLACK_Py " : DataStoreRead  DataStoreName=BLACK_Py  IndexOptions=Index vector (dialog)  Indices=1  OutputSizes=1
  BLACK_Rz : DataStoreRead  DataStoreName=BLACK_Rz  IndexOptions=Index vector (dialog)  Indices=1  OutputSizes=1
  BLACK_RzD : Subsystem  Commented=on
  BLACK_RzD1 : Subsystem
  BLACK_Tz : DataStoreWrite  DataStoreName=BLACK_Tz  IndexOptions=Index vector (dialog)  Indices=1  OutputSizes=1
  Custom Discrete PD (Attitude) : Subsystem
  Custom Discrete PD (X-Position) : Subsystem
  Custom Discrete PD (Y-Position) : Subsystem
  Data Store Write3 : DataStoreWrite  DataStoreName=Float_State  IndexOptions=Index vector (dialog)  Indices=1  OutputSizes=1
  Desired X-Position (BLACK) : Constant  Value=xLength/2  SampleTime=-1
  Desired Y-Position (BLACK) : Constant  Value=yLength/2  SampleTime=-1
  Hough Control : Subsystem
  Puck State : Constant
  Subtract : Sum  Inputs=+-
  Subtract1 : Sum  Inputs=+-
  wires:
  Puck State/1 -> Data Store Write3/1
  BLACK_Px/1 -> Subtract/2
  Custom Discrete PD (Y-Position)/1(Fy) -> BLACK_Fy/1
  Subtract/1 -> Custom Discrete PD (X-Position)/1(ex)
  Desired Y-Position (BLACK)/1 -> Subtract1/1
  Custom Discrete PD (Attitude)/1(Tz) -> BLACK_Tz/1
  Subtract1/1 -> Custom Discrete PD (Y-Position)/1(ey)
  BLACK_Rz/1 -> Hough Control/2(Act)
  Custom Discrete PD (X-Position)/1(Fx) -> BLACK_Fx/1
  Hough Control/1(Err) -> Custom Discrete PD (Attitude)/1(ez)
  "BLACK_Py "/1 -> Subtract1/2
  Desired X-Position (BLACK)/1 -> Subtract/1
  BLACK_RzD1/1(Out1) -> Hough Control/1(Ref)

== system Template_v3_08_2022a_Jetson/Phase #3: Experiment/Change BLACK Behavior/Subsystem ==
  Universal_Time : DataStoreRead  DataStoreName=Univ_Time  IndexOptions=Index vector (dialog)  Indices=1  OutputSizes=1
  Time : Outport  VectorParamsAs1DForOutWhenUnconnected=off
  wires:
  Universal_Time/1 -> Time/1

== system Template_v3_08_2022a_Jetson/Phase #3: Experiment/Change BLUE Behavior/Sub-Phase #1 ==
  note: PD Control Law - BLUE
  note: A simple PD control law is used here to command the platform to it's initial position, as defined in the initializer.
  note: Additional Blocks
  note: Additional blocks are stored here.
  Action Port : ActionPort  ActionPortLabel=if(u1 < u2)
  BLUE_Fx : DataStoreWrite  DataStoreName=BLUE_Fx  IndexOptions=Index vector (dialog)  Indices=1  OutputSizes=1
  BLUE_Fy : DataStoreWrite  DataStoreName=BLUE_Fy  IndexOptions=Index vector (dialog)  Indices=1  OutputSizes=1
  BLUE_Px : DataStoreRead  DataStoreName=BLUE_Px  IndexOptions=Index vector (dialog)  Indices=1  OutputSizes=1
  "BLUE_Py " : DataStoreRead  DataStoreName=BLUE_Py  IndexOptions=Index vector (dialog)  Indices=1  OutputSizes=1
  BLUE_Rz : DataStoreRead  DataStoreName=BLUE_Rz  IndexOptions=Index vector (dialog)  Indices=1  OutputSizes=1
  BLUE_Tz : DataStoreWrite  DataStoreName=BLUE_Tz  IndexOptions=Index vector (dialog)  Indices=1  OutputSizes=1
  Custom Discrete PD (Attitude) : Subsystem
  Custom Discrete PD (X-Position) : Subsystem
  Custom Discrete PD (Y-Position) : Subsystem
  Data Store Write1 : DataStoreWrite  DataStoreName=Float_State  IndexOptions=Index vector (dialog)  Indices=1  OutputSizes=1
  Hough Control : Subsystem
  MATLAB Function2 : MATLAB Function  TreatAsAtomicUnit=on
  MATLAB Function3 : MATLAB Function  TreatAsAtomicUnit=on
  Puck State : Constant
  RED_Rz_REF1 : Subsystem
  Subsystem2 : Subsystem
  Subtract : Sum  Inputs=+-
  Subtract1 : Sum  Inputs=+-
  wires:
  Puck State/1 -> Data Store Write1/1
  Subtract/1 -> Custom Discrete PD (X-Position)/1(ex)
  Custom Discrete PD (X-Position)/1(Fx) -> BLUE_Fx/1
  Subtract1/1 -> Custom Discrete PD (Y-Position)/1(ey)
  Hough Control/1(Err) -> Custom Discrete PD (Attitude)/1(ez)
  Custom Discrete PD (Attitude)/1(Tz) -> BLUE_Tz/1
  Custom Discrete PD (Y-Position)/1(Fy) -> BLUE_Fy/1
  MATLAB Function3/1(y) -> Subtract1/1
  BLUE_Px/1 -> Subtract/2
  MATLAB Function2/1(x) -> Subtract/1
  Subsystem2/1(Out1) -> MATLAB Function2/1(t), MATLAB Function3/1(t)
  "BLUE_Py "/1 -> Subtract1/2
  RED_Rz_REF1/1(Ref) -> Hough Control/1(Ref)
  BLUE_Rz/1 -> Hough Control/2(Act)

== system Template_v3_08_2022a_Jetson/Phase #3: Experiment/Change BLUE Behavior/Sub-Phase #2  ==
  note: Additional blocks are stored here.
  note: A simple PD control law is used here to command the platform to it's initial position, as defined in the initializer.
  note: Additional Blocks
  note: PD Control Law - BLUE
  Action Port : ActionPort  ActionPortLabel=elseif(u1 < u3)
  BLUE_Fx : DataStoreWrite  DataStoreName=BLUE_Fx  IndexOptions=Index vector (dialog)  Indices=1  OutputSizes=1
  BLUE_Fy : DataStoreWrite  DataStoreName=BLUE_Fy  IndexOptions=Index vector (dialog)  Indices=1  OutputSizes=1
  BLUE_Px : DataStoreRead  DataStoreName=BLUE_Px  IndexOptions=Index vector (dialog)  Indices=1  OutputSizes=1
  "BLUE_Py " : DataStoreRead  DataStoreName=BLUE_Py  IndexOptions=Index vector (dialog)  Indices=1  OutputSizes=1
  BLUE_Rz : DataStoreRead  DataStoreName=BLUE_Rz  IndexOptions=Index vector (dialog)  Indices=1  OutputSizes=1
  BLUE_Tz : DataStoreWrite  DataStoreName=BLUE_Tz  IndexOptions=Index vector (dialog)  Indices=1  OutputSizes=1
  Custom Discrete PD (Attitude) : Subsystem
  Custom Discrete PD (X-Position) : Subsystem
  Custom Discrete PD (Y-Position) : Subsystem
  Data Store Write1 : DataStoreWrite  DataStoreName=Float_State  IndexOptions=Index vector (dialog)  Indices=1  OutputSizes=1
  Hough Control : Subsystem
  MATLAB Function2 : MATLAB Function  TreatAsAtomicUnit=on
  MATLAB Function3 : MATLAB Function  TreatAsAtomicUnit=on
  Puck State : Constant
  RED_Rz_REF1 : Subsystem
  Subsystem2 : Subsystem
  Subtract : Sum  Inputs=+-
  Subtract1 : Sum  Inputs=+-
  wires:
  Puck State/1 -> Data Store Write1/1
  BLUE_Rz/1 -> Hough Control/2(Act)
  RED_Rz_REF1/1(Ref) -> Hough Control/1(Ref)
  Custom Discrete PD (Y-Position)/1(Fy) -> BLUE_Fy/1
  Subtract/1 -> Custom Discrete PD (X-Position)/1(ex)
  Subtract1/1 -> Custom Discrete PD (Y-Position)/1(ey)
  BLUE_Px/1 -> Subtract/2
  Custom Discrete PD (X-Position)/1(Fx) -> BLUE_Fx/1
  "BLUE_Py "/1 -> Subtract1/2
  Subsystem2/1(Out1) -> MATLAB Function2/1(t), MATLAB Function3/1(t)
  MATLAB Function2/1(x) -> Subtract/1
  Hough Control/1(Err) -> Custom Discrete PD (Attitude)/1(ez)
  MATLAB Function3/1(y) -> Subtract1/1
  Custom Discrete PD (Attitude)/1(Tz) -> BLUE_Tz/1

== system Template_v3_08_2022a_Jetson/Phase #3: Experiment/Change BLUE Behavior/Sub-Phase #3  ==
  note: Additional blocks are stored here.
  note: A simple PD control law is used here to command the platform to it's initial position, as defined in the initializer.
  note: Additional Blocks
  note: PD Control Law - BLUE
  Action Port : ActionPort  ActionPortLabel=elseif( u1 < u4)
  BLUE_Fx : DataStoreWrite  DataStoreName=BLUE_Fx  IndexOptions=Index vector (dialog)  Indices=1  OutputSizes=1
  BLUE_Fy : DataStoreWrite  DataStoreName=BLUE_Fy  IndexOptions=Index vector (dialog)  Indices=1  OutputSizes=1
  BLUE_Px : DataStoreRead  DataStoreName=BLUE_Px  IndexOptions=Index vector (dialog)  Indices=1  OutputSizes=1
  "BLUE_Py " : DataStoreRead  DataStoreName=BLUE_Py  IndexOptions=Index vector (dialog)  Indices=1  OutputSizes=1
  BLUE_Rz : DataStoreRead  DataStoreName=BLUE_Rz  IndexOptions=Index vector (dialog)  Indices=1  OutputSizes=1
  BLUE_Tz : DataStoreWrite  DataStoreName=BLUE_Tz  IndexOptions=Index vector (dialog)  Indices=1  OutputSizes=1
  Custom Discrete PD (Attitude) : Subsystem
  Custom Discrete PD (X-Position) : Subsystem
  Custom Discrete PD (Y-Position) : Subsystem
  Data Store Write1 : DataStoreWrite  DataStoreName=Float_State  IndexOptions=Index vector (dialog)  Indices=1  OutputSizes=1
  Hough Control : Subsystem
  MATLAB Function2 : MATLAB Function  TreatAsAtomicUnit=on
  MATLAB Function3 : MATLAB Function  TreatAsAtomicUnit=on
  Puck State : Constant
  RED_Rz_REF1 : Subsystem
  Subsystem2 : Subsystem
  Subtract : Sum  Inputs=+-
  Subtract1 : Sum  Inputs=+-
  wires:
  Puck State/1 -> Data Store Write1/1
  BLUE_Rz/1 -> Hough Control/2(Act)
  RED_Rz_REF1/1(Ref) -> Hough Control/1(Ref)
  Custom Discrete PD (Y-Position)/1(Fy) -> BLUE_Fy/1
  Subtract/1 -> Custom Discrete PD (X-Position)/1(ex)
  Subtract1/1 -> Custom Discrete PD (Y-Position)/1(ey)
  BLUE_Px/1 -> Subtract/2
  Custom Discrete PD (X-Position)/1(Fx) -> BLUE_Fx/1
  "BLUE_Py "/1 -> Subtract1/2
  Subsystem2/1(Out1) -> MATLAB Function2/1(t), MATLAB Function3/1(t)
  MATLAB Function2/1(x) -> Subtract/1
  Hough Control/1(Err) -> Custom Discrete PD (Attitude)/1(ez)
  MATLAB Function3/1(y) -> Subtract1/1
  Custom Discrete PD (Attitude)/1(Tz) -> BLUE_Tz/1

== system Template_v3_08_2022a_Jetson/Phase #3: Experiment/Change BLUE Behavior/Sub-Phase #4 ==
  note: Additional blocks are stored here.
  note: A simple PD control law is used here to command the platform to it's initial position, as defined in the initializer.
  note: Additional Blocks
  note: PD Control Law - BLUE
  Action Port : ActionPort  ActionPortLabel=elseif( u1 < u5)
  BLUE_Fx : DataStoreWrite  DataStoreName=BLUE_Fx  IndexOptions=Index vector (dialog)  Indices=1  OutputSizes=1
  BLUE_Fy : DataStoreWrite  DataStoreName=BLUE_Fy  IndexOptions=Index vector (dialog)  Indices=1  OutputSizes=1
  BLUE_Px : DataStoreRead  DataStoreName=BLUE_Px  IndexOptions=Index vector (dialog)  Indices=1  OutputSizes=1
  "BLUE_Py " : DataStoreRead  DataStoreName=BLUE_Py  IndexOptions=Index vector (dialog)  Indices=1  OutputSizes=1
  BLUE_Rz : DataStoreRead  DataStoreName=BLUE_Rz  IndexOptions=Index vector (dialog)  Indices=1  OutputSizes=1
  BLUE_Tz : DataStoreWrite  DataStoreName=BLUE_Tz  IndexOptions=Index vector (dialog)  Indices=1  OutputSizes=1
  Custom Discrete PD (Attitude) : Subsystem
  Custom Discrete PD (X-Position) : Subsystem
  Custom Discrete PD (Y-Position) : Subsystem
  Data Store Write1 : DataStoreWrite  DataStoreName=Float_State  IndexOptions=Index vector (dialog)  Indices=1  OutputSizes=1
  Hough Control : Subsystem
  MATLAB Function2 : MATLAB Function  TreatAsAtomicUnit=on
  MATLAB Function3 : MATLAB Function  TreatAsAtomicUnit=on
  Puck State : Constant
  RED_Rz_REF1 : Subsystem
  Subsystem2 : Subsystem
  Subtract : Sum  Inputs=+-
  Subtract1 : Sum  Inputs=+-
  wires:
  Puck State/1 -> Data Store Write1/1
  BLUE_Rz/1 -> Hough Control/2(Act)
  RED_Rz_REF1/1(Ref) -> Hough Control/1(Ref)
  Custom Discrete PD (Y-Position)/1(Fy) -> BLUE_Fy/1
  Subtract/1 -> Custom Discrete PD (X-Position)/1(ex)
  Subtract1/1 -> Custom Discrete PD (Y-Position)/1(ey)
  BLUE_Px/1 -> Subtract/2
  Custom Discrete PD (X-Position)/1(Fx) -> BLUE_Fx/1
  "BLUE_Py "/1 -> Subtract1/2
  Subsystem2/1(Out1) -> MATLAB Function2/1(t), MATLAB Function3/1(t)
  MATLAB Function2/1(x) -> Subtract/1
  Hough Control/1(Err) -> Custom Discrete PD (Attitude)/1(ez)
  MATLAB Function3/1(y) -> Subtract1/1
  Custom Discrete PD (Attitude)/1(Tz) -> BLUE_Tz/1

== system Template_v3_08_2022a_Jetson/Phase #3: Experiment/Change BLUE Behavior/Subsystem ==
  Universal_Time : DataStoreRead  DataStoreName=Univ_Time  IndexOptions=Index vector (dialog)  Indices=1  OutputSizes=1
  Time : Outport  VectorParamsAs1DForOutWhenUnconnected=off
  wires:
  Universal_Time/1 -> Time/1

== system Template_v3_08_2022a_Jetson/Phase #3: Experiment/Change RED Behavior/Sub-Phase #1 ==
  note: PD Control Law - RED
  note: Additional Blocks
  note: Additional blocks are stored above. Note that to control attitude using the RW, simply replace RED_Tz with RED_Tz_RW.
  note: A simple PD control law is used here to command the platform to it's initial position, as defined in the initializer.
  note: ARM Control Law - RED
  Action Port : ActionPort  ActionPortLabel=if(u1 < u2)
  Constant1 : Constant  Value=0
  Constant4 : Constant  Value=platformSelection
  Custom Discrete PD (Attitude) : Subsystem
  Custom Discrete PD (X-Position) : Subsystem
  Custom Discrete PD (Y-Position) : Subsystem
  Data Store Write3 : DataStoreWrite  DataStoreName=Float_State  IndexOptions=Index vector (dialog)  Indices=1  OutputSizes=1
  Hough Control : Subsystem
  If : If  IfExpression=u1 == 4 | u1 == 5 | u1 == 10 | u1 == 11
  MATLAB Function : MATLAB Function  TreatAsAtomicUnit=on
  MATLAB Function1 : MATLAB Function  TreatAsAtomicUnit=on
  Puck State : Constant
  RED : Subsystem  TreatAsAtomicUnit=on
  RED+ARM : Subsystem  TreatAsAtomicUnit=on
  RED_Fx : DataStoreWrite  DataStoreName=RED_Fx  IndexOptions=Index vector (dialog)  Indices=1  OutputSizes=1
  RED_Fy : DataStoreWrite  DataStoreName=RED_Fy  IndexOptions=Index vector (dialog)  Indices=1  OutputSizes=1
  RED_Px3 : DataStoreRead  DataStoreName=RED_Px  IndexOptions=Index vector (dialog)  Indices=1  OutputSizes=1
  "RED_Py " : DataStoreRead  DataStoreName=RED_Py  IndexOptions=Index vector (dialog)  Indices=1  OutputSizes=1
  RED_Rz : DataStoreRead  DataStoreName=RED_Rz  IndexOptions=Index vector (dialog)  Indices=1  OutputSizes=1
  RED_RzD : Subsystem
  RED_Tz : DataStoreWrite  DataStoreName=RED_Tz  IndexOptions=Index vector (dialog)  Indices=1  OutputSizes=1
  RED_Tz_RW : DataStoreWrite  DataStoreName=RED_Tz_RW  IndexOptions=Index vector (dialog)  Indices=1  OutputSizes=1
  Subsystem1 : Subsystem
  Subtract : Sum  Inputs=+-
  Subtract1 : Sum  Inputs=+-
  wires:
  Constant1/1 -> RED_Tz_RW/1
  Puck State/1 -> Data Store Write3/1
  Custom Discrete PD (Y-Position)/1(Fy) -> RED_Fy/1
  Custom Discrete PD (X-Position)/1(Fx) -> RED_Fx/1
  Custom Discrete PD (Attitude)/1(Tz) -> RED_Tz/1
  Hough Control/1(Err) -> Custom Discrete PD (Attitude)/1(ez)
  Subsystem1/1(Out1) -> MATLAB Function/1(t), MATLAB Function1/1(t)
  RED_Px3/1 -> Subtract/2
  MATLAB Function1/1(y) -> Subtract1/1
  "RED_Py "/1 -> Subtract1/2
  MATLAB Function/1(x) -> Subtract/1
  Subtract/1 -> Custom Discrete PD (X-Position)/1(ex)
  RED_Rz/1 -> Hough Control/2(Act)
  Subtract1/1 -> Custom Discrete PD (Y-Position)/1(ey)
  RED_RzD/1(Ref) -> Hough Control/1(Ref)
  If/1 -> RED+ARM/Action
  Constant4/1 -> If/1
  If/2 -> RED/Action

== system Template_v3_08_2022a_Jetson/Phase #3: Experiment/Change RED Behavior/Sub-Phase #2  ==
  note: PD Control Law - RED
  note: Additional Blocks
  note: Additional blocks are stored above. Note that to control attitude using the RW, simply replace RED_Tz with RED_Tz_RW.
  note: ARM Control Law - RED
  Action Port : ActionPort  ActionPortLabel=elseif(u1 < u3)
  BLACK_RzD1 : Subsystem
  Constant1 : Constant  Value=0
  Constant4 : Constant  Value=platformSelection
  Custom Discrete PD (Attitude) : Subsystem
  Custom Discrete PD (X-Position) : Subsystem
  Custom Discrete PD (Y-Position) : Subsystem
  Data Store Write3 : DataStoreWrite  DataStoreName=Float_State  IndexOptions=Index vector (dialog)  Indices=1  OutputSizes=1
  Hough Control : Subsystem
  If : If  IfExpression=u1 == 4 | u1 == 5 | u1 == 10 | u1 == 11
  MATLAB Function : MATLAB Function  TreatAsAtomicUnit=on
  MATLAB Function1 : MATLAB Function  TreatAsAtomicUnit=on
  Puck State : Constant
  RED : Subsystem  TreatAsAtomicUnit=on
  RED+ARM : Subsystem  TreatAsAtomicUnit=on
  RED_Fx : DataStoreWrite  DataStoreName=RED_Fx  IndexOptions=Index vector (dialog)  Indices=1  OutputSizes=1
  RED_Fy : DataStoreWrite  DataStoreName=RED_Fy  IndexOptions=Index vector (dialog)  Indices=1  OutputSizes=1
  RED_Px1 : DataStoreRead  DataStoreName=RED_Px  IndexOptions=Index vector (dialog)  Indices=1  OutputSizes=1
  "RED_Py " : DataStoreRead  DataStoreName=RED_Py  IndexOptions=Index vector (dialog)  Indices=1  OutputSizes=1
  RED_Rz : DataStoreRead  DataStoreName=RED_Rz  IndexOptions=Index vector (dialog)  Indices=1  OutputSizes=1
  RED_Tz : DataStoreWrite  DataStoreName=RED_Tz  IndexOptions=Index vector (dialog)  Indices=1  OutputSizes=1
  RED_Tz_RW : DataStoreWrite  DataStoreName=RED_Tz_RW  IndexOptions=Index vector (dialog)  Indices=1  OutputSizes=1
  Subsystem1 : Subsystem
  Subtract : Sum  Inputs=+-
  Subtract2 : Sum  Inputs=+-
  wires:
  Constant1/1 -> RED_Tz_RW/1
  Puck State/1 -> Data Store Write3/1
  Subtract2/1 -> Custom Discrete PD (Y-Position)/1(ey)
  "RED_Py "/1 -> Subtract2/2
  BLACK_RzD1/1(Ref) -> Hough Control/1(Ref)
  MATLAB Function/1(x) -> Subtract/1
  RED_Rz/1 -> Hough Control/2(Act)
  Subtract/1 -> Custom Discrete PD (X-Position)/1(ex)
  MATLAB Function1/1(y) -> Subtract2/1
  Custom Discrete PD (Attitude)/1(Tz) -> RED_Tz/1
  RED_Px1/1 -> Subtract/2
  Subsystem1/1(Out1) -> MATLAB Function/1(t), MATLAB Function1/1(t)
  Custom Discrete PD (X-Position)/1(Fx) -> RED_Fx/1
  Hough Control/1(Err) -> Custom Discrete PD (Attitude)/1(ez)
  Custom Discrete PD (Y-Position)/1(Fy) -> RED_Fy/1
  If/1 -> RED+ARM/Action
  Constant4/1 -> If/1
  If/2 -> RED/Action

== system Template_v3_08_2022a_Jetson/Phase #3: Experiment/Change RED Behavior/Sub-Phase #3  ==
  note: PD Control Law - RED
  note: Additional Blocks
  note: Additional blocks are stored above. Note that to control attitude using the RW, simply replace RED_Tz with RED_Tz_RW.
  note: ARM Control Law - RED
  Action Port : ActionPort  ActionPortLabel=elseif( u1 < u4)
  Constant1 : Constant  Value=platformSelection
  Constant4 : Constant  Value=0
  Custom Discrete PD (Attitude) : Subsystem  Commented=on
  Custom Discrete PD (X-Position) : Subsystem
  Custom Discrete PD (Y-Position) : Subsystem
  Data Store Write3 : DataStoreWrite  DataStoreName=Float_State  IndexOptions=Index vector (dialog)  Indices=1  OutputSizes=1
  Hough Control : Subsystem  Commented=on
  If : If  IfExpression=u1 == 4 | u1 == 5 | u1 == 10 | u1 == 11
  MATLAB Function : MATLAB Function  TreatAsAtomicUnit=on
  MATLAB Function1 : MATLAB Function  TreatAsAtomicUnit=on
  Puck State : Constant
  RED : Subsystem  TreatAsAtomicUnit=on
  RED+ARM : Subsystem  TreatAsAtomicUnit=on
  RED_Fx : DataStoreWrite  DataStoreName=RED_Fx  IndexOptions=Index vector (dialog)  Indices=1  OutputSizes=1
  RED_Fy : DataStoreWrite  DataStoreName=RED_Fy  IndexOptions=Index vector (dialog)  Indices=1  OutputSizes=1
  RED_Px1 : DataStoreRead  DataStoreName=RED_Px  IndexOptions=Index vector (dialog)  Indices=1  OutputSizes=1
  "RED_Py " : DataStoreRead  DataStoreName=RED_Py  IndexOptions=Index vector (dialog)  Indices=1  OutputSizes=1
  RED_Rz : DataStoreRead  Commented=on  DataStoreName=RED_Rz  IndexOptions=Index vector (dialog)  Indices=1  OutputSizes=1
  RED_Rz_REF : Subsystem  Commented=on
  RED_Tz : DataStoreWrite  Commented=on  DataStoreName=RED_Tz  IndexOptions=Index vector (dialog)  Indices=1  OutputSizes=1
  RED_Tz_RW : DataStoreWrite  DataStoreName=RED_Tz_RW  IndexOptions=Index vector (dialog)  Indices=1  OutputSizes=1
  Saturation : Saturate  UpperLimit=Tz_lim_sharm  LowerLimit=-Tz_lim_sharm
  Saturation1 : Saturate  UpperLimit=Tz_lim_elarm  LowerLimit=-Tz_lim_elarm
  Saturation3 : Saturate  UpperLimit=Tz_lim_wrarm  LowerLimit=-Tz_lim_wrarm
  Subsystem1 : Subsystem
  Subtract : Sum  Inputs=+-
  Subtract2 : Sum  Inputs=+-
  wires:
  Puck State/1 -> Data Store Write3/1
  Hough Control/1(Err) -> Custom Discrete PD (Attitude)/1(ez)
  Custom Discrete PD (Y-Position)/1(Fy) -> RED_Fy/1
  Custom Discrete PD (X-Position)/1(Fx) -> RED_Fx/1
  RED_Rz/1 -> Hough Control/2(Act)
  MATLAB Function1/1(y) -> Subtract2/1
  Custom Discrete PD (Attitude)/1(Tz) -> RED_Tz/1
  MATLAB Function/1(x) -> Subtract/1
  Subtract/1 -> Custom Discrete PD (X-Position)/1(ex)
  "RED_Py "/1 -> Subtract2/2
  RED_Rz_REF/1(Ref) -> Hough Control/1(Ref)
  RED_Px1/1 -> Subtract/2
  Subsystem1/1(Out1) -> MATLAB Function/1(t), MATLAB Function1/1(t)
  Subtract2/1 -> Custom Discrete PD (Y-Position)/1(ey)
  Constant4/1 -> RED_Tz_RW/1
  If/1 -> RED+ARM/Action
  Constant1/1 -> If/1
  If/2 -> RED/Action
